simulink model "Ship_location_model_simulation_final"  (R2024b)
settings: Solver=VariableStepAuto  StartTime=0.0  StopTime=50  RelTol=1e-3
libraries: simulink x3
settings Model: Creator=danie  LastModifiedBy=danie
settings SolverCC: AlgebraicLoopSolver=TrustRegion
settings RTWCC: DLArmComputeVersion=19.05

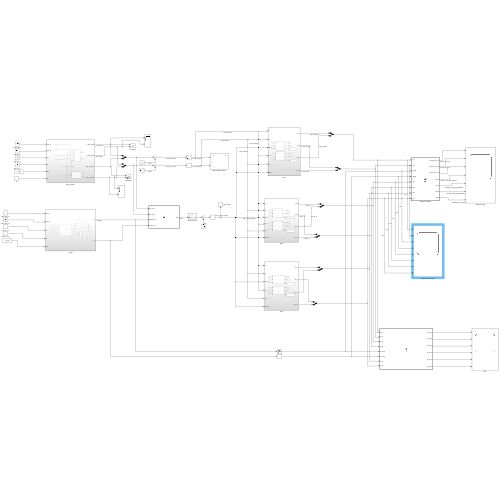
[thumbnail: Simulink's stored preview of the top-level diagram]
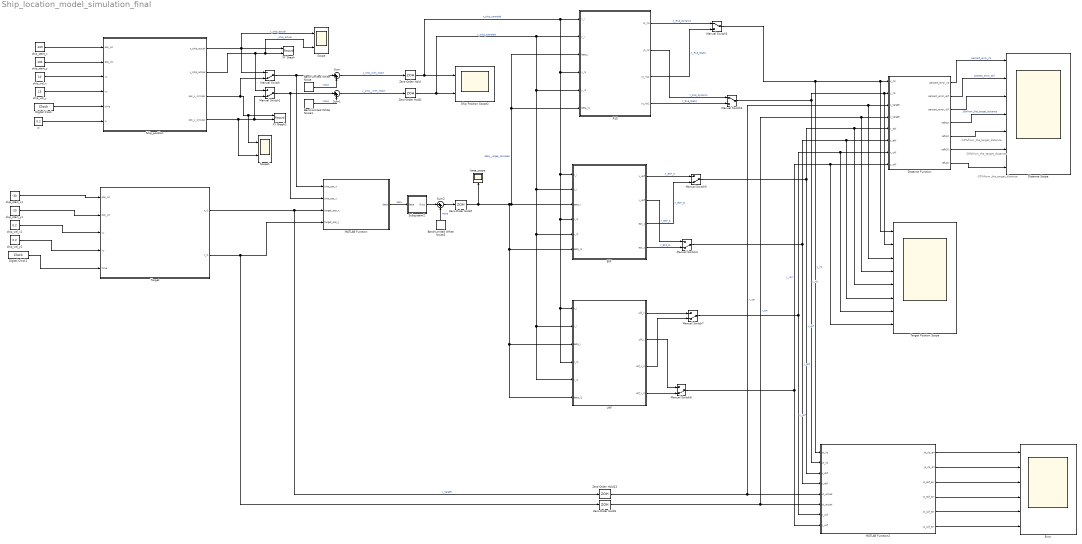
== system Ship_location_model_simulation_final ==
  note: -20%from_the_target_distance
  note: 20%from_the_target_distance
  note: -10%from_the_target_distance
  Band-Limited White Noise : simulink/Sources/Band-Limited White Noise  Cov=[1]  Ts=0.1  seed=[23341]
  Band-Limited White Noise1 : simulink/Sources/Band-Limited White Noise  Cov=[1]  Ts=0.1  seed=[233471]
  Band-Limited White Noise2 : simulink/Sources/Band-Limited White Noise  Cov=[ 0.1900e-05]  Ts=0.01  seed=[21113341]
  Digital Clock : DigitalClock  SampleTime=0.1
  Digital Clock1 : DigitalClock  SampleTime=0.1
  Distance Function : MATLAB Function  TreatAsAtomicUnit=on
  Distance Scope : Scope  NumInputPorts=7
  EKF : Subsystem
  Error : Scope  NumInputPorts=6
      settings: Description=error
  MATLAB Function : MATLAB Function  TreatAsAtomicUnit=on
  MATLAB Function2 : MATLAB Function  TreatAsAtomicUnit=on
  Manual Switch{,1,4..7} (6 alike) : ManualSwitch  CurrentSetting=0
  Manual Switch2 : ManualSwitch
  Manual Switch3 : ManualSwitch
  RLS : Subsystem
  Scope : Scope  NumInputPorts=2
  Scope1 : Scope  NumInputPorts=2
  Ship Position Scope2 : Scope  NumInputPorts=2
  Ship_position : Subsystem
  Subsystem2 : Subsystem
  Sum : Sum  Inputs=|++
  Sum1 : Sum  Inputs=|++
  Sum2 : Sum  Inputs=|++
  Target : Subsystem
  Target Position Scope : Scope  NumInputPorts=8
  UKF : Subsystem
  XY Graph : Record  FileSettingsInternal="{\"entries\":[{\"content\":{\"excelSettings\":{\"content\":{},\"type\":\"Streamout.ExcelSettings\"}},\"type\":\"Streamout.FileSettingStorage\",\"uuid\":\"\"}],\"packageUris\":[\"http:\\/\\/schema.mathworks.com\\/mf0\\/streamout_blocks\\/R2020a\"],\"version\":\"1.0\"}"  Layout=[1 1]  SignalsInternal="{\"entries\":[{\"content\":{\"signals\":[{\"content\":{\"blockPath\":[],\"dimensions\":[1],\"domain\":\"\",\"lineColor\":\"#a2142f\",\"plots\":[ 1 ],\"port\":1,\"sid\":[\"\"],\"signalID\":1,\"signalName\":\"x_ship_actual\"},\"type\":\"RecordBlkView.Signal\",\"uuid\":\"\"},{\"content\":{\"blockPath\":[],\"dimensions\":[1],\"domain\":\"\",\"lineColor\":\"#139fff\",\"plots\":[ 1 ],\"port\":2,\"sid\":[\"\"],\"signalID\":2,\"signalName\":\"_ship_actual\"},\"type\":\"RecordBlkView.Signal\",\"uuid\":\"\"}]},\"type\":\"RecordBlkView.InputSignals\",\"uuid\":\"\"}],\"packageUris\":[\"http:\\/\\/schema.mathworks.com\\/mf0\\/streamout_blocks\\/R2020a\"],\"version\":\"1.0\"}"  VisualizationBindings="{\"xyplotplugin\":{\"info\":[{\"series\":[{\"bindingParametersList\":[{\"parameter\":\"X-Axis\",\"signalID\":1,\"signalName\":\"x_ship_actual\"},{\"parameter\":\"Y-Axis\",\"signalID\":2,\"signalName\":\"_ship_actual\"}],\"seriesID\":0}],\"subplotID\":1}]}}"  CompatibilityTag=XY
  XY Graph1 : Record  FileSettingsInternal="{\"entries\":[{\"content\":{\"excelSettings\":{\"content\":{},\"type\":\"Streamout.ExcelSettings\"}},\"type\":\"Streamout.FileSettingStorage\",\"uuid\":\"\"}],\"packageUris\":[\"http:\\/\\/schema.mathworks.com\\/mf0\\/streamout_blocks\\/R2020a\"],\"version\":\"1.0\"}"  Layout=[1 1]  SignalsInternal="{\"entries\":[{\"content\":{\"signals\":[{\"content\":{\"blockPath\":[],\"dimensions\":[1],\"domain\":\"\",\"lineColor\":\"#a2142f\",\"plots\":[ 1 ],\"port\":1,\"sid\":[\"\"],\"signalID\":1,\"signalName\":\"Ship_position:3\"},\"type\":\"RecordBlkView.Signal\",\"uuid\":\"\"},{\"content\":{\"blockPath\":[],\"dimensions\":[1],\"domain\":\"\",\"lineColor\":\"#139fff\",\"plots\":[ 1 ],\"port\":2,\"sid\":[\"\"],\"signalID\":2,\"signalName\":\"Ship_position:4\"},\"type\":\"RecordBlkView.Signal\",\"uuid\":\"\"}]},\"type\":\"RecordBlkView.InputSignals\",\"uuid\":\"\"}],\"packageUris\":[\"http:\\/\\/schema.mathworks.com\\/mf0\\/streamout_blocks\\/R2020a\"],\"version\":\"1.0\"}"  VisualizationBindings="{\"xyplotplugin\":{\"info\":[{\"series\":[{\"bindingParametersList\":[{\"parameter\":\"X-Axis\",\"signalID\":1,\"signalName\":\"Ship_position:3\"},{\"parameter\":\"Y-Axis\",\"signalID\":2,\"signalName\":\"Ship_position:4\"}],\"seriesID\":0}],\"subplotID\":1}]}}"  CompatibilityTag=XY
  Zero-Order Hold : ZeroOrderHold  SampleTime=0.01
  Zero-Order Hold1 : ZeroOrderHold  SampleTime=0.01
  Zero-Order Hold13 : ZeroOrderHold
  Zero-Order Hold2 : ZeroOrderHold  SampleTime=0.01
  Zero-Order Hold3 : ZeroOrderHold
  beta_scope : Scope
  ship_start_x : Constant  Value=-100
  ship_start_x1 : Constant  Value=-30
  ship_start_y : Constant  Value=100
  ship_start_y1 : Constant  Value=-25
  ship_vel_x : Constant  Value=10
  ship_vel_x1 : Constant  Value=0.2
  ship_vel_y : Constant  Value=15
  ship_vel_y1 : Constant  Value=0.2
  w : Constant  Value=0.2
  wires:
  ship_start_x/1 -> Ship_position/1(pos_x0)
  ship_start_y/1 -> Ship_position/2(pos_y0)
  ship_vel_x/1 -> Ship_position/3(vx)
  ship_vel_y/1 -> Ship_position/4(vy)
  Digital Clock/1 -> Ship_position/5(time)
  w/1 -> Ship_position/6(w)
  Band-Limited White Noise/1 -> Sum/2  "noise"
  Sum/1 -> Zero-Order Hold/1  "x_ship_with_noise"
  Band-Limited White Noise1/1 -> Sum1/2  "noise"
  Zero-Order Hold1/1 -> UKF/5(y_i1), UKF/2(y_i), EKF/5(y_i1), EKF/2(y_i), RLS/5(y_i1), RLS/2(y_i), Ship Position Scope2/2  "y_ship_sampled"
  Sum1/1 -> Zero-Order Hold1/1  "y_ship__with_noise"
  Zero-Order Hold/1 -> EKF/1(x_i), UKF/4(x_i1), UKF/1(x_i), EKF/4(x_i1), RLS/4(x_i1), RLS/1(x_i), Ship Position Scope2/1  "x_ship_sampled"
  Ship_position/3(pos_x_circular) -> Manual Switch/2, XY Graph1/1, Scope1/1
  Ship_position/1(x_ship_actual) -> XY Graph/1, Scope/1, Manual Switch/1  "x_ship_actual"
  Ship_position/2(y_ship_actual) -> Manual Switch1/1, XY Graph/2, Scope/2  "_ship_actual"
  Ship_position/4(pos_y_circular) -> Scope1/2, XY Graph1/2, Manual Switch1/2
  Manual Switch/1 -> MATLAB Function/1(ship_pos_x), Sum/1
  Manual Switch1/1 -> MATLAB Function/2(ship_pos_y), Sum1/1
  ship_start_x1/1 -> Target/1(pos_x0)
  ship_start_y1/1 -> Target/2(pos_y0)
  Sum2/1 -> Zero-Order Hold2/1
  Band-Limited White Noise2/1 -> Sum2/2  "noise"
  Zero-Order Hold2/1 -> EKF/3(beta_i), RLS/6(beta_i1), RLS/3(beta_i), UKF/3(beta_i), UKF/6(beta_i1), EKF/6(beta_i1), beta_scope/1  "beta__angel_sampled"
  RLS/3(xt_rls1) -> Manual Switch3/2  "X_RLS_Static"
  RLS/1(xt_rls) -> Manual Switch3/1  "X_RLS_Dynamic"
  EKF/3(est_x) -> Manual Switch5/2  "X_EKF_D"
  EKF/1(x_ekf) -> Manual Switch5/1  "X_EKF_S"
  EKF/4(est_y) -> Manual Switch4/2  "Y_EKF_D"
  EKF/2(y_ekf) -> Manual Switch4/1  "Y_EKF_S"
  UKF/1(ukf_x) -> Manual Switch7/1
  UKF/3(ukf_x_2) -> Manual Switch7/2
  UKF/2(ukf_y) -> Manual Switch6/1
  UKF/4(ukf_y_2) -> Manual Switch6/2
  RLS/4(yt_rls1) -> Manual Switch2/2  "Y_RLS_Static"
  RLS/2(yt_rls) -> Manual Switch2/1  "Y_RLS_Dynamic"
  Manual Switch5/1 -> MATLAB Function2/3(x_ekf), Target Position Scope/5, Distance Function/5(x_ekf)  "x_ekf"
  Manual Switch2/1 -> Target Position Scope/2, Distance Function/2(y_rls), MATLAB Function2/2(yt_rls)  "y_rls"
  Manual Switch3/1 -> MATLAB Function2/1(xt_rls), Target Position Scope/1, Distance Function/1(x_rls)  "x_rls"
  MATLAB Function2/1(xt_rls_err) -> Error/1
  MATLAB Function2/2(yt_rls_err) -> Error/2
  MATLAB Function2/3(xt_ekf_err) -> Error/3
  MATLAB Function2/4(yt_ekf_err) -> Error/4
  MATLAB Function2/5(xt_ukf_err) -> Error/5
  MATLAB Function2/6(yt_ukf_err) -> Error/6
  Zero-Order Hold13/1 -> Target Position Scope/3, Distance Function/3(x_target), MATLAB Function2/5(xt_actual)  "x_tar"
  Zero-Order Hold3/1 -> Target Position Scope/4, Distance Function/4(y_target), MATLAB Function2/6(yt_actual)  "y_tar"
  Manual Switch4/1 -> Target Position Scope/6, Distance Function/6(y_ekf), MATLAB Function2/4(y_ekf)  "y_ekf"
  Manual Switch7/1 -> Target Position Scope/7, Distance Function/7(x_ukf), MATLAB Function2/7(x_ukf)  "x_ukf"
  Manual Switch6/1 -> Target Position Scope/8, Distance Function/8(y_ukf), MATLAB Function2/8(y_ukf)  "y_ukf"
  Distance Function/4(refH10) -> Distance Scope/4  "10%from_the_target_distance"
  Distance Function/3(percent_error_ukf) -> Distance Scope/3
  Distance Function/2(percent_error_ekf) -> Distance Scope/2  "precent_error_ekf"
  Distance Function/1(percent_error_rls) -> Distance Scope/1  "percent_error_rls"
  ship_vel_x1/1 -> Target/3(vx)
  Digital Clock1/1 -> Target/5(time)
  ship_vel_y1/1 -> Target/4(vy)
  Target/1(x_i1) -> Zero-Order Hold13/1, MATLAB Function/3(target_pos_x)  "x_target"
  Target/2(y_i1) -> Zero-Order Hold3/1, MATLAB Function/4(target_pos_y)
  Distance Function/5(refL10) -> Distance Scope/5
  Distance Function/6(refH20) -> Distance Scope/6
  Distance Function/7(refL20) -> Distance Scope/7
  MATLAB Function/1(beta) -> Subsystem2/1(beta)  "beta"
  Subsystem2/1(Out1) -> Sum2/1

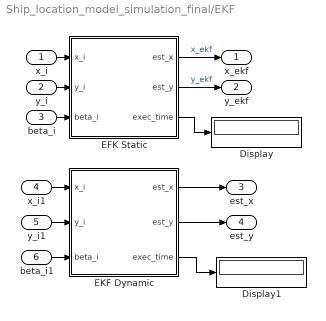
== system Ship_location_model_simulation_final/EKF ==
  x_i : Inport
  y_i : Inport  Port=2
  beta_i : Inport  Port=3
  x_i1 : Inport  Port=4
  y_i1 : Inport  Port=5
  beta_i1 : Inport  Port=6
  Display : Display
  Display1 : Display
  EFK Static : MATLAB Function  TreatAsAtomicUnit=on
  EKF Dynamic : MATLAB Function  TreatAsAtomicUnit=on
  x_ekf : Outport
  y_ekf : Outport  Port=2
  est_x : Outport  Port=3
  est_y : Outport  Port=4
  wires:
  y_i/1 -> EFK Static/2(y_i)
  EKF Dynamic/2(est_y) -> est_y/1
  x_i/1 -> EFK Static/1(x_i)
  x_i1/1 -> EKF Dynamic/1(x_i)
  y_i1/1 -> EKF Dynamic/2(y_i)
  EFK Static/2(est_y) -> y_ekf/1  "y_ekf"
  EFK Static/1(est_x) -> x_ekf/1  "x_ekf"
  beta_i/1 -> EFK Static/3(beta_i)
  beta_i1/1 -> EKF Dynamic/3(beta_i)
  EKF Dynamic/1(est_x) -> est_x/1
  EFK Static/3(exec_time) -> Display/1
  EKF Dynamic/3(exec_time) -> Display1/1

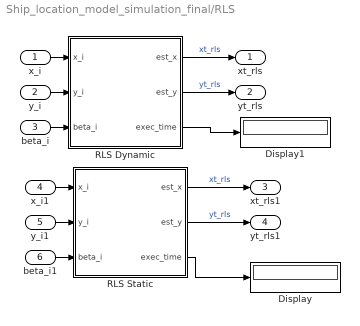
== system Ship_location_model_simulation_final/RLS ==
  x_i : Inport
  y_i : Inport  Port=2
  beta_i : Inport  Port=3
  x_i1 : Inport  Port=4
  y_i1 : Inport  Port=5
  beta_i1 : Inport  Port=6
  Display : Display
  Display1 : Display
  RLS Dynamic : MATLAB Function  TreatAsAtomicUnit=on
  RLS Static : MATLAB Function  TreatAsAtomicUnit=on
  xt_rls : Outport
  yt_rls : Outport  Port=2
  xt_rls1 : Outport  Port=3
  yt_rls1 : Outport  Port=4
  wires:
  RLS Static/1(est_x) -> xt_rls1/1  "xt_rls"
  beta_i/1 -> RLS Dynamic/3(beta_i)
  y_i1/1 -> RLS Static/2(y_i)
  x_i1/1 -> RLS Static/1(x_i)
  beta_i1/1 -> RLS Static/3(beta_i)
  x_i/1 -> RLS Dynamic/1(x_i)
  RLS Static/2(est_y) -> yt_rls1/1  "yt_rls"
  y_i/1 -> RLS Dynamic/2(y_i)
  RLS Dynamic/1(est_x) -> xt_rls/1  "xt_rls"
  RLS Dynamic/2(est_y) -> yt_rls/1  "yt_rls"
  RLS Static/3(exec_time) -> Display/1
  RLS Dynamic/3(exec_time) -> Display1/1

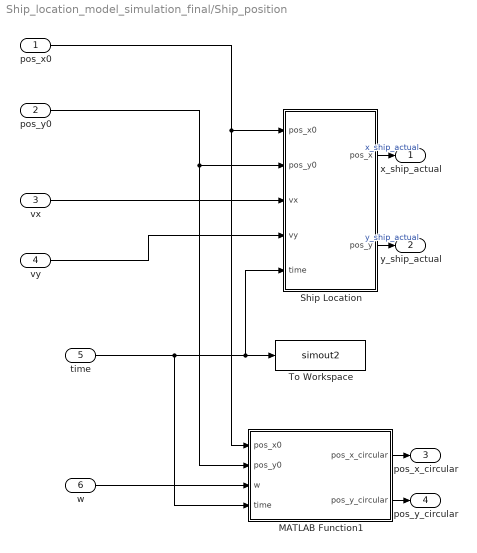
== system Ship_location_model_simulation_final/Ship_position ==
  pos_x0 : Inport
  pos_y0 : Inport  Port=2
  vx : Inport  Port=3
  vy : Inport  Port=4
  time : Inport  Port=5
  w : Inport  Port=6
  MATLAB Function1 : MATLAB Function  TreatAsAtomicUnit=on
  Ship Location : MATLAB Function  TreatAsAtomicUnit=on
  To Workspace : ToWorkspace  VariableName=simout2  SaveFormat=Timeseries  SampleTime=-1
  x_ship_actual : Outport
  y_ship_actual : Outport  Port=2
  pos_x_circular : Outport  Port=3
  pos_y_circular : Outport  Port=4
  wires:
  vx/1 -> Ship Location/3(vx)
  time/1 -> MATLAB Function1/4(time), Ship Location/5(time), To Workspace/1
  pos_y0/1 -> MATLAB Function1/2(pos_y0), Ship Location/2(pos_y0)
  pos_x0/1 -> MATLAB Function1/1(pos_x0), Ship Location/1(pos_x0)
  Ship Location/1(pos_x) -> x_ship_actual/1  "x_ship_actual"
  MATLAB Function1/2(pos_y_circular) -> pos_y_circular/1
  vy/1 -> Ship Location/4(vy)
  w/1 -> MATLAB Function1/3(w)
  MATLAB Function1/1(pos_x_circular) -> pos_x_circular/1
  Ship Location/2(pos_y) -> y_ship_actual/1  "y_ship_actual"

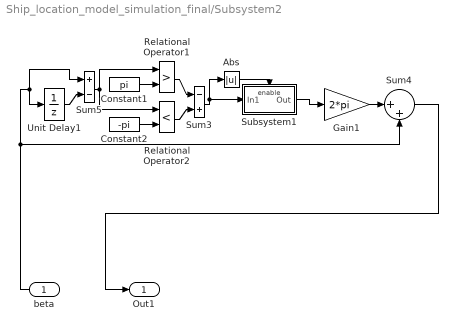
== system Ship_location_model_simulation_final/Subsystem2 ==
  beta : Inport
  Abs : Abs
  Constant1 : Constant  Value=pi
  Constant2 : Constant  Value=-pi
  Gain1 : Gain  Gain=2*pi  SaturateOnIntegerOverflow=on  OutDataTypeStr=Inherit: Same as input  ParamDataTypeStr=Inherit: Same as input
  Relational Operator1 : RelationalOperator  Operator=>  InputSameDT=off
  Relational Operator2 : RelationalOperator  Operator=<  InputSameDT=off
  Subsystem1 : Subsystem
  Sum3 : Sum  Inputs=-+  OutDataTypeStr=double  SaturateOnIntegerOverflow=on
  Sum4 : Sum  Inputs=|++  SaturateOnIntegerOverflow=on
  Sum5 : Sum  Inputs=+-  SaturateOnIntegerOverflow=on
  Unit Delay1 : UnitDelay  SampleTime=0.01  HasFrameUpgradeWarning=on
  Out1 : Outport
  wires:
  Constant2/1 -> Relational Operator2/2
  Sum5/1 -> Relational Operator1/1, Relational Operator2/1
  Unit Delay1/1 -> Sum5/2
  Relational Operator2/1 -> Sum3/2
  Gain1/1 -> Sum4/1
  beta/1 -> Sum5/1, Unit Delay1/1, Sum4/2
  Relational Operator1/1 -> Sum3/1
  Sum3/1 -> Subsystem1/1(In1), Abs/1
  Subsystem1/1(Out) -> Gain1/1
  Constant1/1 -> Relational Operator1/2
  Abs/1 -> Subsystem1/Enable
  Sum4/1 -> Out1/1

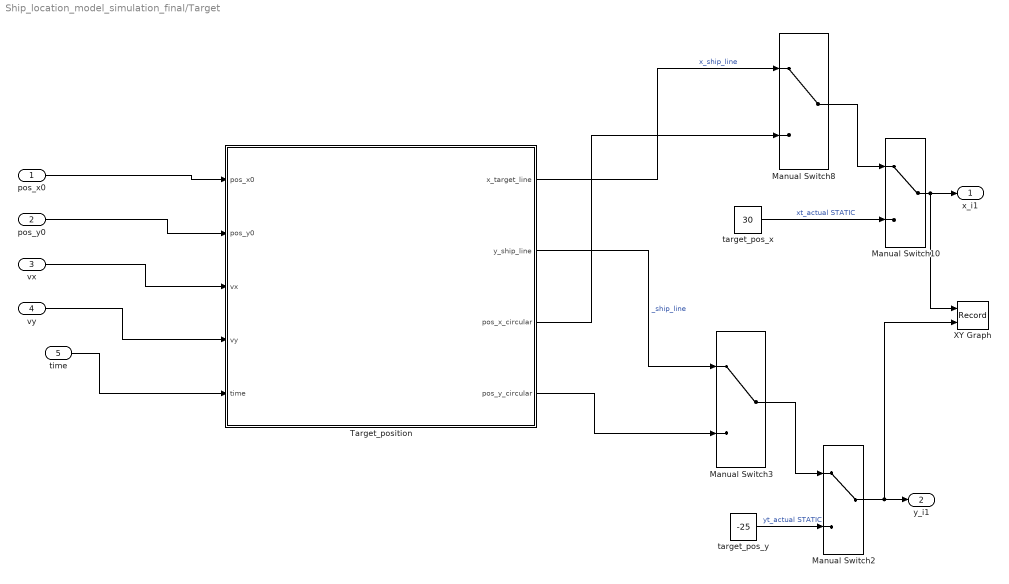
== system Ship_location_model_simulation_final/Target ==
  pos_x0 : Inport
  pos_y0 : Inport  Port=2
  vx : Inport  Port=3
  vy : Inport  Port=4
  time : Inport  Port=5
  Manual Switch{2..3,8,10} (4 alike) : ManualSwitch
  Target_position : Subsystem
  XY Graph : Record  FileSettingsInternal="{\"entries\":[{\"content\":{\"excelSettings\":{\"content\":{},\"type\":\"Streamout.ExcelSettings\"}},\"type\":\"Streamout.FileSettingStorage\",\"uuid\":\"\"}],\"packageUris\":[\"http:\\/\\/schema.mathworks.com\\/mf0\\/streamout_blocks\\/R2020a\"],\"version\":\"1.0\"}"  Layout=[1 1]  SignalsInternal="{\"entries\":[{\"content\":{\"signals\":[{\"content\":{\"blockPath\":[],\"dimensions\":[1],\"domain\":\"\",\"lineColor\":\"#a2142f\",\"plots\":[ 1 ],\"port\":1,\"sid\":[\"\"],\"signalID\":1,\"signalName\":\"Manual Switch10\"},\"type\":\"RecordBlkView.Signal\",\"uuid\":\"\"},{\"content\":{\"blockPath\":[],\"dimensions\":[1],\"domain\":\"\",\"lineColor\":\"#139fff\",\"plots\":[ 1 ],\"port\":2,\"sid\":[\"\"],\"signalID\":2,\"signalName\":\"Manual Switch2\"},\"type\":\"RecordBlkView.Signal\",\"uuid\":\"\"}]},\"type\":\"RecordBlkView.InputSignals\",\"uuid\":\"\"}],\"packageUris\":[\"http:\\/\\/schema.mathworks.com\\/mf0\\/streamout_blocks\\/R2020a\"],\"version\":\"1.0\"}"  VisualizationBindings="{\"xyplotplugin\":{\"info\":[{\"series\":[{\"bindingParametersList\":[{\"parameter\":\"X-Axis\",\"signalID\":1,\"signalName\":\"Manual Switch10\"},{\"parameter\":\"Y-Axis\",\"signalID\":2,\"signalName\":\"Manual Switch2\"}],\"seriesID\":0}],\"subplotID\":1}]}}"  CompatibilityTag=XY
  target_pos_x : Constant  Value=30
  target_pos_y : Constant  Value=-25
  x_i1 : Outport
  y_i1 : Outport  Port=2
  wires:
  Target_position/3(pos_x_circular) -> Manual Switch8/2
  target_pos_y/1 -> Manual Switch2/2  "yt_actual STATIC"
  Target_position/4(pos_y_circular) -> Manual Switch3/2
  Target_position/2(y_ship_line) -> Manual Switch3/1  "_ship_line"
  Manual Switch10/1 -> XY Graph/1, x_i1/1
  Manual Switch8/1 -> Manual Switch10/1
  vx/1 -> Target_position/3(vx)
  Manual Switch3/1 -> Manual Switch2/1
  Target_position/1(x_target_line) -> Manual Switch8/1  "x_ship_line"
  target_pos_x/1 -> Manual Switch10/2  "xt_actual STATIC"
  pos_x0/1 -> Target_position/1(pos_x0)
  Manual Switch2/1 -> XY Graph/2, y_i1/1
  pos_y0/1 -> Target_position/2(pos_y0)
  time/1 -> Target_position/5(time)
  vy/1 -> Target_position/4(vy)

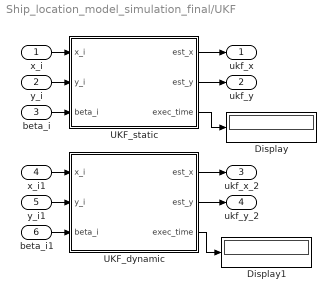
== system Ship_location_model_simulation_final/UKF ==
  x_i : Inport
  y_i : Inport  Port=2
  beta_i : Inport  Port=3
  x_i1 : Inport  Port=4
  y_i1 : Inport  Port=5
  beta_i1 : Inport  Port=6
  Display : Display
  Display1 : Display
  UKF_dynamic : MATLAB Function  TreatAsAtomicUnit=on
  UKF_static : MATLAB Function  TreatAsAtomicUnit=on
  ukf_x : Outport
  ukf_y : Outport  Port=2
  ukf_x_2 : Outport  Port=3
  ukf_y_2 : Outport  Port=4
  wires:
  UKF_dynamic/1(est_x) -> ukf_x_2/1
  UKF_static/2(est_y) -> ukf_y/1
  beta_i/1 -> UKF_static/3(beta_i)
  x_i/1 -> UKF_static/1(x_i)
  x_i1/1 -> UKF_dynamic/1(x_i)
  UKF_static/1(est_x) -> ukf_x/1
  y_i1/1 -> UKF_dynamic/2(y_i)
  y_i/1 -> UKF_static/2(y_i)
  UKF_dynamic/2(est_y) -> ukf_y_2/1
  beta_i1/1 -> UKF_dynamic/3(beta_i)
  UKF_static/3(exec_time) -> Display/1
  UKF_dynamic/3(exec_time) -> Display1/1

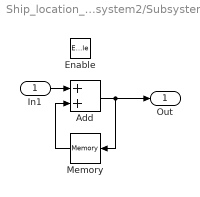
== system Ship_location_model_simulation_final/Subsystem2/Subsystem1 ==
  In1 : Inport
  Enable : EnablePort
  Add : Sum
  Memory : Memory
  Out : Outport
  wires:
  Memory/1 -> Add/2
  Add/1 -> Out/1, Memory/1
  In1/1 -> Add/1

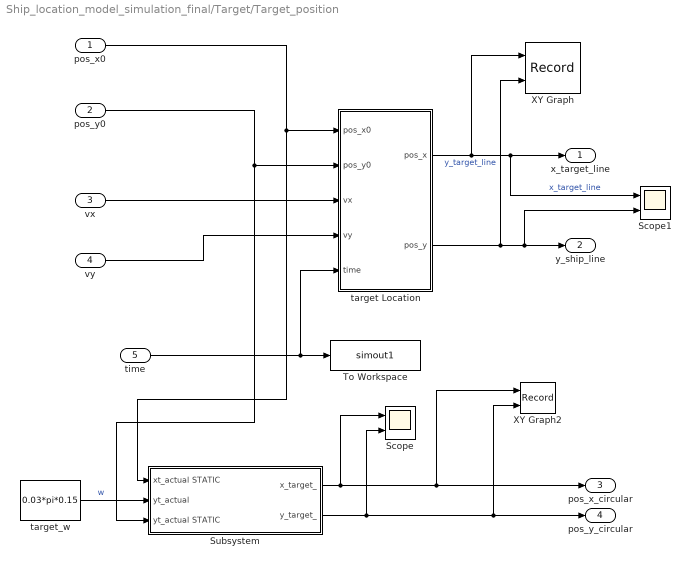
== system Ship_location_model_simulation_final/Target/Target_position ==
  pos_x0 : Inport
  pos_y0 : Inport  Port=2
  vx : Inport  Port=3
  vy : Inport  Port=4
  time : Inport  Port=5
  Scope : Scope  NumInputPorts=2
  Scope1 : Scope  NumInputPorts=2
  Subsystem : Subsystem
  To Workspace : ToWorkspace  VariableName=simout1  SaveFormat=Timeseries  SampleTime=-1
  XY Graph : Record  FileSettingsInternal="{\"entries\":[{\"content\":{\"excelSettings\":{\"content\":{},\"type\":\"Streamout.ExcelSettings\"}},\"type\":\"Streamout.FileSettingStorage\",\"uuid\":\"\"}],\"packageUris\":[\"http:\\/\\/schema.mathworks.com\\/mf0\\/streamout_blocks\\/R2020a\"],\"version\":\"1.0\"}"  Layout=[1 1]  SignalsInternal="{\"entries\":[{\"content\":{\"signals\":[{\"content\":{\"blockPath\":[],\"dimensions\":[1],\"domain\":\"\",\"lineColor\":\"#22b573\",\"lineWidth\":2,\"port\":1,\"sid\":[\"\"],\"signalID\":1,\"signalName\":\"x_target_line\"},\"type\":\"RecordBlkView.Signal\",\"uuid\":\"\"},{\"content\":{\"blockPath\":[],\"dimensions\":[1],\"domain\":\"\",\"lineColor\":\"#0072bd\",\"lineWidth\":2,\"port\":2,\"sid\":[\"\"],\"signalID\":2,\"signalName\":\"y_target_line\"},\"type\":\"RecordBlkView.Signal\",\"uuid\":\"\"}]},\"type\":\"RecordBlkView.InputSignals\",\"uuid\":\"\"}],\"packageUris\":[\"http:\\/\\/schema.mathworks.com\\/mf0\\/streamout_blocks\\/R2020a\"],\"version\":\"1.0\"}"  VisualizationBindings="{\"xyplotplugin\":{\"info\":[{\"series\":[],\"subplotID\":1}]}}"  CompatibilityTag=XY  st=-1
  XY Graph2 : Record  FileSettingsInternal="{\"entries\":[{\"content\":{\"excelSettings\":{\"content\":{},\"type\":\"Streamout.ExcelSettings\"}},\"type\":\"Streamout.FileSettingStorage\",\"uuid\":\"\"}],\"packageUris\":[\"http:\\/\\/schema.mathworks.com\\/mf0\\/streamout_blocks\\/R2020a\"],\"version\":\"1.0\"}"  Layout=[1 1]  SignalsInternal="{\"entries\":[{\"content\":{\"signals\":[{\"content\":{\"blockPath\":[],\"dimensions\":[1],\"domain\":\"\",\"lineColor\":\"#d95319\",\"lineWidth\":2,\"port\":1,\"sid\":[\"\"],\"signalID\":1,\"signalName\":\"Subsystem:1\"},\"type\":\"RecordBlkView.Signal\",\"uuid\":\"\"},{\"content\":{\"blockPath\":[],\"dimensions\":[1],\"domain\":\"\",\"lineColor\":\"#edb120\",\"lineWidth\":2,\"port\":2,\"sid\":[\"\"],\"signalID\":2,\"signalName\":\"Subsystem:2\"},\"type\":\"RecordBlkView.Signal\",\"uuid\":\"\"}]},\"type\":\"RecordBlkView.InputSignals\",\"uuid\":\"\"}],\"packageUris\":[\"http:\\/\\/schema.mathworks.com\\/mf0\\/streamout_blocks\\/R2020a\"],\"version\":\"1.0\"}"  CompatibilityTag=XY
  target Location : MATLAB Function  TreatAsAtomicUnit=on
  target_w : Constant  Value=0.03*pi*0.15
  x_target_line : Outport
  y_ship_line : Outport  Port=2
  pos_x_circular : Outport  Port=3
  pos_y_circular : Outport  Port=4
  wires:
  vx/1 -> target Location/3(vx)
  time/1 -> target Location/5(time), To Workspace/1
  pos_y0/1 -> Subsystem/3(yt_actual STATIC), target Location/2(pos_y0)
  pos_x0/1 -> Subsystem/1(xt_actual STATIC), target Location/1(pos_x0)
  target Location/1(pos_x) -> XY Graph/1, Scope1/1, x_target_line/1  "x_target_line"
  Subsystem/2(y_target_) -> Scope/2, XY Graph2/2, pos_y_circular/1
  vy/1 -> target Location/4(vy)
  Subsystem/1(x_target_) -> Scope/1, XY Graph2/1, pos_x_circular/1
  target Location/2(pos_y) -> XY Graph/2, Scope1/2, y_ship_line/1  "y_target_line"
  target_w/1 -> Subsystem/2(yt_actual)  "w"

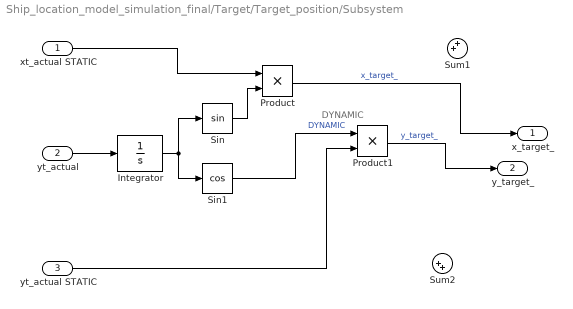
== system Ship_location_model_simulation_final/Target/Target_position/Subsystem ==
  note: DYNAMIC
  xt_actual STATIC : Inport
  yt_actual : Inport  Port=2
  yt_actual STATIC : Inport  Port=3
  Integrator : Integrator
  Product : Product
  Product1 : Product
  Sin : Trigonometry
  Sin1 : Trigonometry  Operator=cos
  Sum1 : Sum  Inputs=++|
  Sum2 : Sum  Inputs=|++
  x_target_ : Outport
  y_target_ : Outport  Port=2
  wires:
  Product1/1 -> y_target_/1  "y_target_"
  Sin/1 -> Product/2
  Integrator/1 -> Sin/1, Sin1/1
  Sin1/1 -> Product1/1  "DYNAMIC"
  Product/1 -> x_target_/1  "x_target_"
  yt_actual/1 -> Integrator/1
  xt_actual STATIC/1 -> Product/1
  yt_actual STATIC/1 -> Product1/2

== matlab function Ship_location_model_simulation_final/RLS/RLS Static ==
  data: x_i input; est_x output; y_i input; beta_i input; est_y output; exec_time output
function [est_x, est_y, exec_time] = fcn(x_i, y_i, beta_i)  
% FCN Perform recursive estimation for position using a RLS algorithm  
% Outputs:  
% - est_x: Estimated x-coordinate  
% - est_y: Estimated y-coordinate  
% - exec_time: Execution time (fixed-size double for Simulink compatibility)  

% Declare persistent variables  
persistent Q P X_i  

% Initialize execution time variable  
exec_time = 0; % Explicitly define as a scalar double (important for Simulink)  

% Start timing  
coder.extrinsic('tic', 'toc'); % Allow tic/toc in Simulink  
tStart = tic; % Capture start time  

% Initialization of the covariance matrix P on the first function call  
if isempty(P)  
    P = 1000 * eye(2); % Start with a large initial uncertainty  
end  

if isempty(Q)  
    Q = 0 * eye(2); % No process noise initially  
end  

% Initialization of the state vector X_i on the first function call  
if isempty(X_i)  
    X_i = zeros(2, 1); % Start with zero state  
end  

% Observation vector based on the angle beta_i  
phi_i = [-sin(beta_i); cos(beta_i)]; % The observation model  

% Measurement scalar z_i derived from the input coordinates and angle  
z_i = y_i * cos(beta_i) - x_i * sin(beta_i);  

% The estimation error  
e = z_i - phi_i' * X_i; % Prediction error  

% The weighting vector  
g_k = P * phi_i / (1 + phi_i' * P * phi_i);  

% Update the state vector with the new measurement  
X_i = X_i + g_k * e;  

% Update the covariance matrix  
P = P - g_k * phi_i' * P + Q;  

% Extract estimated position  
est_x = X_i(1);  
est_y = X_i(2);  

% End timing and store execution time  
exec_time = toc(tStart); % Ensure exec_time is a fixed-size double  

end

== matlab function Ship_location_model_simulation_final/Distance Function ==
  data: percent_error_rls output; percent_error_ekf output; percent_error_ukf output; x_rls input; refH10 output; y_rls input; x_target input; y_target input; x_ekf input; y_ekf input; x_ukf input; y_ukf input; refL10 output; refH20 output; refL20 output
function [percent_error_rls,percent_error_ekf,percent_error_ukf,refH10, refL10,refH20, refL20]= fcn(x_rls,y_rls,x_target,y_target, x_ekf, y_ekf,x_ukf, y_ukf)
% Outputs:
%   percent_error_rls - Percentage error in distance for the RLS estimate
%   percent_error_ekf - Percentage error in distance for the EKF estimate
%   ref - Reference value defined as 10% of the target distance

% The Euclidean distance for the RLS estimate
distance_rls = sqrt(x_rls^2 + y_rls^2);

% The Euclidean distance for the EKF estimate
distance_ekf = sqrt(x_ekf^2 + y_ekf^2);

% The Euclidean distance to the actual target
distance_target = sqrt(x_target^2 + y_target^2);

% The distance percentage error for the RLS estimation
percent_error_rls = ((distance_rls - distance_target) / distance_target) * 100;

% The distance percentage error for the EKF estimation
percent_error_ekf = ((distance_ekf - distance_target) / distance_target) * 100;

% The reference value as 10% of the target distance
refH10 = 0.1 * distance_target;
refL10 = -0.1 * distance_target;

refH20 = 0.2 * distance_target;
refL20 = -0.2 * distance_target;

distance_ukf = sqrt(x_ukf^2 + y_ukf^2);
percent_error_ukf = ((distance_ukf - distance_target) / distance_target) * 100;


end

== matlab function Ship_location_model_simulation_final/MATLAB Function2 ==
  data: xt_rls input; xt_rls_err output; yt_rls_err output; yt_rls input; x_ekf input; y_ekf input; xt_actual input; yt_actual input; xt_ekf_err output; yt_ekf_err output; x_ukf input; y_ukf input; xt_ukf_err output; yt_ukf_err output
function [xt_rls_err,yt_rls_err,xt_ekf_err,yt_ekf_err,xt_ukf_err,yt_ukf_err]   = fcn(xt_rls,yt_rls, x_ekf, y_ekf,xt_actual,yt_actual,x_ukf,y_ukf)
% FCN Computes the percentage error for RLS and EKF position estimates

% The percentage error for RLS estimates:
xt_rls_err = ((xt_rls - xt_actual)/xt_actual)*100;
yt_rls_err = ((yt_rls - yt_actual)/yt_actual)*100;

% The percentage error for EKF estimates:
xt_ekf_err = ((x_ekf - xt_actual)/xt_actual)*100;
yt_ekf_err = ((y_ekf - yt_actual)/yt_actual)*100;

xt_ukf_err = ((x_ukf - xt_actual)/xt_actual)*100;
yt_ukf_err = ((y_ukf - yt_actual)/yt_actual)*100;

== matlab function Ship_location_model_simulation_final/UKF/UKF_static ==
  data: x_i input; est_x output; y_i input; beta_i input; est_y output; exec_time output
function [est_x, est_y, exec_time] = ukf_fcn(x_i, y_i, beta_i)

persistent X_i P Q R lambda alpha beta nx

% Initialize execution time variable  
exec_time = 0; % Ensures fixed-size output for Simulink compatibility  

% Start timing  
coder.extrinsic('tic', 'toc'); % Allows tic/toc in Simulink  
tStart = tic; % Capture start time 

if isempty(P)
    nx = 6; % State dimension
    P = 1000* eye(nx); % Covariance matrix initialization (6x6)
    Q = 0.001 * diag([0.01, 0.01, 1, 0.01, 1, 0.01]); % Process noise covariance (6x6)
    R = diag([1, 1, 100]); % Measurement noise covariance (3x3)
    
    % UKF parameters
    alpha = 1e-3; % Spread of sigma points
    beta = 2; % Optimal for Gaussian distribution
    lambda = alpha^2 * (nx + 1) - nx; % Scaling parameter
end

if isempty(X_i)
    X_i = zeros(nx, 1); % State vector initialization (6x1)
end

dt = 0.01; % Sample time variable

% Weights for UKF
Wm = [lambda / (nx + lambda); repmat(1 / (2 * (nx + lambda)), 2 * nx, 1)];
Wc = Wm;
Wc(1) = Wc(1) + (1 - alpha^2 + beta);

% Generate sigma points
sigma_points = generate_sigma_points(X_i, P, lambda);

% Prediction Step
predicted_sigma_points = process_model(sigma_points, dt);
[X_pred, P_pred] = compute_mean_and_covariance(predicted_sigma_points, Wm, Wc, Q);

% Measurement Step
measured_sigma_points = measurement_model(predicted_sigma_points, beta_i);
[y_pred, Pyy] = compute_mean_and_covariance(measured_sigma_points, Wm, Wc, R);

% Cross covariance
Pxy = compute_cross_covariance(predicted_sigma_points, measured_sigma_points, X_pred, y_pred, Wc);

% Kalman Gain
K = Pxy / Pyy;

% Measurement update
meas = [x_i; y_i; 0]; % Measurements
resid = meas - y_pred; % Residual
X_i = X_pred + K * resid; % State update
P = P_pred - K * Pyy * K'; % Covariance update

% Output estimated position
est_x = X_i(1); % x_t estimation
est_y = X_i(2); % y_t estimation

% Stop timing  
exec_time = toc(tStart); % Store execution time

end

%% Helper Functions

% Generate sigma points
function sigma_points = generate_sigma_points(mean, covariance, lambda)
    nx = length(mean);
    S = chol((nx + lambda) * covariance, 'lower');
    sigma_points = [mean, bsxfun(@plus, mean, S), bsxfun(@minus, mean, S)];
end

% Process model
function predicted_sigma_points = process_model(sigma_points, dt)
    F = [1 0 0 0 0 0;
         0 1 0 0 0 0;
         0 0 1 dt 0 0;
         0 0 0 1 0 0;
         0 0 0 0 1 dt;
         0 0 0 0 0 1]; % Process model matrix
    predicted_sigma_points = F * sigma_points;
end

% Measurement model
function measured_sigma_points = measurement_model(sigma_points, beta_i)
    H = [0 0 1 0 0 0;
         0 0 0 0 1 0;
         sin(beta_i) -cos(beta_i) -sin(beta_i) 0 cos(beta_i) 0]; % Measurement model matrix
    measured_sigma_points = H * sigma_points;
end

% Compute mean and covariance
function [mean_out, covariance] = compute_mean_and_covariance(sigma_points, Wm, Wc, noise_cov)
    mean_out = sigma_points * Wm; % Weighted mean
    diff = bsxfun(@minus, sigma_points, mean_out);
    covariance = diff * diag(Wc) * diff' + noise_cov; % Weighted covariance
end

% Compute cross covariance
function Pxy = compute_cross_covariance(predicted_sigma_points, measured_sigma_points, X_pred, y_pred, Wc)
    diff_x = bsxfun(@minus, predicted_sigma_points, X_pred);
    diff_y = bsxfun(@minus, measured_sigma_points, y_pred);
    Pxy = diff_x * diag(Wc) * diff_y'; % Cross covariance
end

== matlab function Ship_location_model_simulation_final/UKF/UKF_dynamic ==
  data: x_i input; est_x output; y_i input; beta_i input; est_y output; exec_time output
function [est_x, est_y, exec_time] = ukf_dynamic_fcn(x_i, y_i, beta_i)

persistent X_i P Q R lambda alpha beta nx

% Initialize execution time variable  
exec_time = 0; % Ensures fixed-size output for Simulink compatibility  

% Start timing  
coder.extrinsic('tic', 'toc'); % Allows tic/toc in Simulink  
tStart = tic; % Capture start time  

if isempty(P)
    nx = 8; % State dimension for dynamic model
    P = 10 * eye(nx); % Covariance matrix initialization (8x8)
    Q = 0.01 * diag([0.01, 0.01, 1, 0.01, 1, 0.01, 1, 0.01]); % Process noise covariance (8x8)
    R = diag([1, 1, 400]); % Measurement noise covariance (3x3)
    
    % UKF parameters
    alpha = 1e-3; % Spread of sigma points
    beta = 2; % Optimal for Gaussian distribution
    lambda = alpha^2 * (nx + 1) - nx; % Scaling parameter
end

if isempty(X_i)
    X_i = zeros(nx, 1); % State vector initialization (8x1)
end

dt = 0.001; % Sample time variable

% Weights for UKF
Wm = [lambda / (nx + lambda); repmat(1 / (2 * (nx + lambda)), 2 * nx, 1)];
Wc = Wm;
Wc(1) = Wc(1) + (1 - alpha^2 + beta);

% Generate sigma points
sigma_points = generate_sigma_points(X_i, P, lambda);

% Prediction Step
predicted_sigma_points = process_model(sigma_points, dt);
[X_pred, P_pred] = compute_mean_and_covariance(predicted_sigma_points, Wm, Wc, Q);

% Measurement Step
measured_sigma_points = measurement_model(predicted_sigma_points, beta_i);
[y_pred, Pyy] = compute_mean_and_covariance(measured_sigma_points, Wm, Wc, R);

% Cross covariance
Pxy = compute_cross_covariance(predicted_sigma_points, measured_sigma_points, X_pred, y_pred, Wc);

% Kalman Gain
K = Pxy / Pyy;

% Measurement update
meas = [x_i; y_i; 0]; % Measurements
resid = meas - y_pred; % Residual
X_i = X_pred + K * resid; % State update
P = P_pred - K * Pyy * K'; % Covariance update

% Output estimated position
est_x = X_i(1); % x_t estimation
est_y = X_i(3); % y_t estimation

% Stop timing  
exec_time = toc(tStart); % Store execution time  

end

%% Helper Functions

% Generate sigma points
function sigma_points = generate_sigma_points(mean, covariance, lambda)
    nx = length(mean);
    S = chol((nx + lambda) * covariance, 'lower');
    sigma_points = [mean, bsxfun(@plus, mean, S), bsxfun(@minus, mean, S)];
end

% Process model
function predicted_sigma_points = process_model(sigma_points, dt)
    F = [1 dt 0 0 0 0 0 0; 
         0 1 0 0 0 0 0 0; 
         0 0 1 dt 0 0 0 0; 
         0 0 0 1 0 0 0 0; 
         0 0 0 0 1 dt 0 0; 
         0 0 0 0 0 1 0 0; 
         0 0 0 0 0 0 1 dt; 
         0 0 0 0 0 0 0 1]; % Process model matrix for dynamic system
    predicted_sigma_points = F * sigma_points;
end

% Measurement model
function measured_sigma_points = measurement_model(sigma_points, beta_i)
    H = [0 0 0 0 1 0 0 0;
         0 0 0 0 0 0 1 0;
         sin(beta_i) 0 -cos(beta_i) 0 -sin(beta_i) 0 cos(beta_i) 0]; % Measurement model matrix
    measured_sigma_points = H * sigma_points;
end

% Compute mean and covariance
function [mean_out, covariance] = compute_mean_and_covariance(sigma_points, Wm, Wc, noise_cov)
    mean_out = sigma_points * Wm; % Weighted mean
    diff = bsxfun(@minus, sigma_points, mean_out);
    covariance = diff * diag(Wc) * diff' + noise_cov; % Weighted covariance
end

% Compute cross covariance
function Pxy = compute_cross_covariance(predicted_sigma_points, measured_sigma_points, X_pred, y_pred, Wc)
    diff_x = bsxfun(@minus, predicted_sigma_points, X_pred);
    diff_y = bsxfun(@minus, measured_sigma_points, y_pred);
    Pxy = diff_x * diag(Wc) * diff_y'; % Cross covariance
end

== matlab function Ship_location_model_simulation_final/Ship_position/Ship Location ==
  data: pos_x0 input; pos_x output; pos_y0 input; vx input; vy input; time input; pos_y output
function [pos_x,pos_y] = fcn(pos_x0,pos_y0,vx,vy,time)
% FCN Calculate the position of an object in a 2D plane over time
%
% Inputs:
%   pos_x0 - Initial x-coordinate of the object
%   pos_y0 - Initial y-coordinate of the object
%   vx - Velocity of the object along the x-axis (constant)
%   vy - Velocity of the object along the y-axis (constant)
%   time - Time duration for which the object has been in motion
%
% Outputs:
%   pos_x - Final x-coordinate of the object after the given time
%   pos_y - Final y-coordinate of the object after the given time

% Calculation of the x-coordinate, using the equation of motion
pos_x = vx*time + pos_x0;
% Calculation of the y-coordinate,using the equation of motion
pos_y = vy*time + pos_y0;

== matlab function Ship_location_model_simulation_final/Target/Target_position/target Location ==
  data: pos_x0 input; pos_x output; pos_y0 input; vx input; vy input; time input; pos_y output
function [pos_x,pos_y] = fcn(pos_x0,pos_y0,vx,vy,time)
% FCN Calculate the position of an object in a 2D plane over time
%
% Inputs:
%   pos_x0 - Initial x-coordinate of the object
%   pos_y0 - Initial y-coordinate of the object
%   vx - Velocity of the object along the x-axis (constant)
%   vy - Velocity of the object along the y-axis (constant)
%   time - Time duration for which the object has been in motion
%
% Outputs:
%   pos_x - Final x-coordinate of the object after the given time
%   pos_y - Final y-coordinate of the object after the given time

% Calculation of the x-coordinate, using the equation of motion
pos_x = vx*time + pos_x0;
% Calculation of the y-coordinate,using the equation of motion
pos_y = vy*time + pos_y0;

== matlab function Ship_location_model_simulation_final/Ship_position/MATLAB Function1 ==
  data: pos_x0 input; pos_x_circular output; pos_y0 input; w input; time input; pos_y_circular output
function [pos_x_circular,pos_y_circular] = fcn(pos_x0,pos_y0,w,time)
% FCN Calculate the position of an object moving in a circular path
%
% Inputs:
%   pos_x0 - Initial x-coordinate of the object
%   pos_y0 - Initial y-coordinate of the object
%   w - Angular velocity (rad/s)
%
% Outputs:
%   pos_x_circular - x-coordinate of the object after the given time
%   pos_y_circular - y-coordinate of the object after the given time

% Calculation of the radius of the circular motion
R = sqrt(pos_x0^2+pos_y0^2);

% Calculation of the x-coordinate for circular motion
pos_x_circular = R*cos(w*time) + pos_x0;
% Calculation of the y-coordinate for circular motion
pos_y_circular = R*sin(w*time) + pos_y0;

== matlab function Ship_location_model_simulation_final/MATLAB Function ==
  data: ship_pos_x input; beta output; ship_pos_y input; target_pos_x input; target_pos_y input
function beta = fcn(ship_pos_x,ship_pos_y,target_pos_x,target_pos_y)
% Calculation of the horizontal distance (dx) between the target and the ship

% Calculation of the horizontal distance (dx) between the target and the ship
dx = target_pos_x - ship_pos_x;

% Calculation of the vertical distance (dy) between the target and the ship
dy = target_pos_y - ship_pos_y;

% `atan2(dy, dx)` returns the angle in radians in the range [-pi, pi]
beta = atan2(dy,dx);

end

== matlab function Ship_location_model_simulation_final/EKF/EFK Static ==
  data: x_i input; est_x output; y_i input; beta_i input; est_y output; exec_time output
function [est_x, est_y, exec_time] = ekf_fcn(x_i, y_i, beta_i)

persistent X_i P Q R

% Initialize execution time variable  
exec_time = 0; % Ensures fixed-size output for Simulink compatibility  

% Start timing  
coder.extrinsic('tic', 'toc'); % Allows tic/toc in Simulink  
tStart = tic; % Capture start time

if isempty(P)
    P = 1000*eye(6); % Covariance matrix initialization (6x6)
    Q = 0.001*diag([0.01, 0.01, 1, 0.01, 1, 0.01]); % Process noise covariance initialization (6x6)
    R = diag([1, 1, 100]); % Measurement noise covariance initialization (3x3)
end

if isempty(X_i)
    X_i = zeros(6, 1); % State vector initialization (6x1)
end

dt = 0.01; % Sample time variable
F = [1 0 0 0 0 0 ; 0 1 0 0 0 0 ; 0 0 1 dt 0 0 ; 0 0 0 1 0 0 ; 0 0 0 0 1 dt ; 0 0 0 0 0 1]; % Process Jacobian (6x6)
H = [0 0 1 0 0 0 ; 0 0 0 0 1 0 ; sin(beta_i) -cos(beta_i) -sin(beta_i) 0 cos(beta_i) 0]; % Measurement Jacobian (3x6)

% Prediction Step
X_i = F*X_i; % Process Model
meas = [x_i ; y_i ; 0]; % Measurements
y_hat = H*X_i; % Measurement Model
P = F*P*F' + Q; % Covariance matrix

% Update Step
resid = meas - y_hat; % Measurement residual
K = P*H'/(H*P*H' + R); % Kalman gain
X_i = X_i + K*resid; % State vector update
P = (eye(6) - K*H)*P; % Covariance matrix update

% Output estimated position
est_x = X_i(1); % x_t estimation
est_y = X_i(2); % y_t estimation

% Stop timing  
exec_time = toc(tStart); % Store execution time  

end

== matlab function Ship_location_model_simulation_final/EKF/EKF Dynamic ==
  data: x_i input; est_x output; y_i input; beta_i input; est_y output; exec_time output
function [est_x, est_y, exec_time] = ekf_fcn(x_i, y_i, beta_i)

persistent X_i P Q R

% Initialize execution time variable  
exec_time = 0; % Ensures fixed-size output for Simulink compatibility  

% Start timing  
coder.extrinsic('tic', 'toc'); % Allows tic/toc in Simulink  
tStart = tic; % Capture start time  

if isempty(P)
    P = 10*eye(8); % Covariance matrix initialization (8x8)
    Q = 0.01*diag([0.01, 0.01, 1, 0.01, 1, 0.01, 1, 0.01]); % Process noise covariance initialization (8x8)
    R = diag([1, 1, 400]); % Measurement noise covariance initialization (3x3)
end
 
if isempty(X_i)
    X_i = zeros(8, 1); % State vector initialization (8x1)
end

dt = 0.001; % Sample time variable
F = [1 dt 0 0 0 0 0 0 ; 0 1 0 0 0 0 0 0 ; 0 0 1 dt 0 0 0 0 ; 0 0 0 1 0 0 0 0 ; 0 0 0 0 1 dt 0 0 ; 0 0 0 0 0 1 0 0 ; 0 0 0 0 0 0 1 dt ; 0 0 0 0 0 0 0 1]; % Process Jacobian (8x8)
H = [0 0 0 0 1 0 0 0 ; 0 0 0 0 0 0 1 0 ; sin(beta_i) 0 -cos(beta_i) 0 -sin(beta_i) 0 cos(beta_i) 0]; % Measurement Jacobian (3x8)

% Prediction Step
X_i = F*X_i; % Process Model
meas = [x_i ; y_i ; 0]; % Measurements
y_hat = H*X_i; % Measurement Model
P = F*P*F' + Q; % Covariance matrix

% Update Step
resid = meas - y_hat; % Measurement residual
K = P*H'/(H*P*H' + R); % Kalman gain
X_i = X_i + K*resid; % State vector update
P = (eye(8) - K*H)*P; % Covariance matrix update

% Output estimated position
est_x = X_i(1); % x_t estimation
est_y = X_i(3); % y_t estimation

% Stop timing  
exec_time = toc(tStart); % Store execution time  

end

== matlab function Ship_location_model_simulation_final/RLS/RLS Dynamic ==
  settings: updateMethod=DISCRETE
  data: x_i input; est_x output; y_i input; beta_i input; est_y output; exec_time output
function [est_x, est_y, exec_time] = fcn(x_i, y_i, beta_i) 
% FCN Perform recursive least squares (RLS) algorithm with a forgetting factor to estimate
% the position of a target based on noisy measurements and angular data.
% Outputs: est_x - Estimated x-coordinate of the target and est_y - Estimated y-coordinate of the target

% Declartion of the persistent variables 
persistent P X_i lambda lambda_initial

% Initialize execution time variable  
exec_time = 0; % Ensures fixed-size output for Simulink compatibility  

% Start timing  
coder.extrinsic('tic', 'toc'); % Allows tic/toc in Simulink  
tStart = tic; % Capture start time 

% Initialization of the persistent variables on the first function call
if isempty(P)
    P = 1*eye(2);  % Initialization of the covariance matrix as a 2x2 identity matrix
    lambda_initial = 0.98; % Initial forgetting factor
    lambda = 1; % Initial adaptive forgetting factor
end

if isempty(X_i)
    X_i = zeros(2, 1);  % Initialization of the state vector (X) as a 2x1 zero vector
end

% Update the observation model
phi_i = [-sin(beta_i); cos(beta_i)];  % The observation vector (phi)
z_i = y_i * cos(beta_i) - x_i * sin(beta_i);  % The measurement scalar (z)

% The estimation error
e = z_i - phi_i' * X_i;  % Error between measurement and model prediction

% The weighting vector
g_k = P * phi_i / (lambda + phi_i' * P * phi_i);  

% Updating the state vector with the new measurement
X_i = X_i + g_k * e;  % Recursive state update

% Updating the covariance matrix using the forgetting factor
P = (1 / lambda) * (P - g_k * phi_i' * P);  % Update covariance matrix

% Adapt the forgetting factor
lambda = lambda_initial * lambda + (1 - lambda_initial);

%The estimated position from the updated state vector
est_x = X_i(1);  % Estimated x-coordinate
est_y = X_i(2);  % Estimated y-coordinate

% Stop timing  
exec_time = toc(tStart); % Store execution time  

end
